simulink model "Lyapunov_3d"  (R2014a)
settings: Solver=ode45  StartTime=0.0  StopTime=100  RelTol=1e-3
values from neighbouring files (symbols this model uses):
  beta = 5    [lyapunov_vf.m]    (also in lyapunov_vf_3d.m; vector_cr_1.m)
  gam = 0.2    [lyapunov_vf.m]    (also in lyapunov_vf_3d.m; vector_cr_1.m)
  r = 20    [lsl.m]    (also in lyapunov_vf.m = 30; lyapunov_vf_3d.m = 100; rsl.m)
  vel = 10    [lyapunov_vf.m]    (also in lyapunov_vf_3d.m; vector_cr_1.m)
  x_int = -100    [lsl.m]    (also in lyapunov_vf.m; lyapunov_vf_3d.m = 20; rsl.m = -300; vf.m = 0)
  y_int = 10    [lsl.m]    (also in lyapunov_vf.m = -200; lyapunov_vf_3d.m = 20; rsl.m = 0; vf.m = -50)
  z_int = 10    [lyapunov_vf_3d.m]
settings Model: Creator=User  LastModifiedBy=User

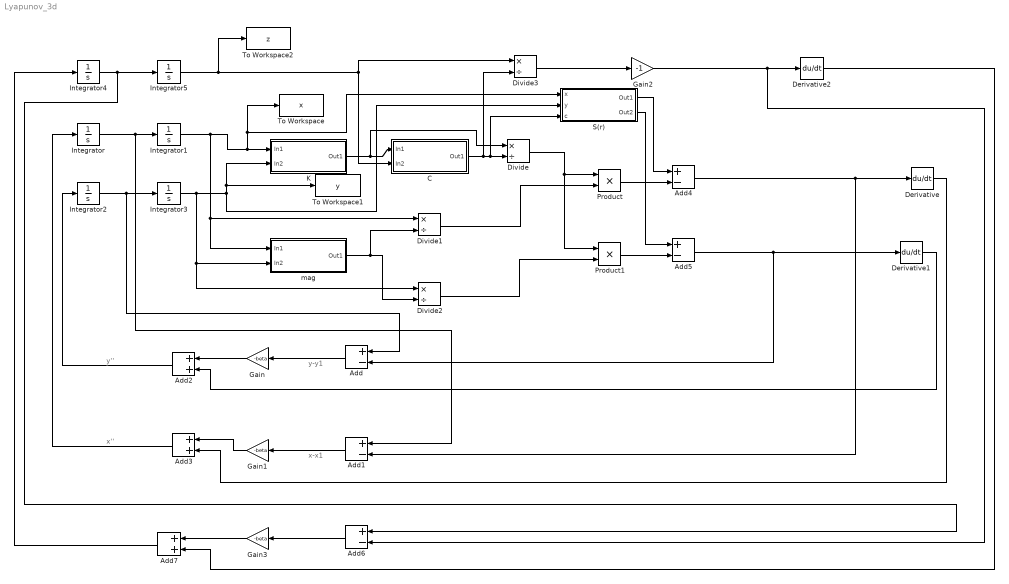
== system Lyapunov_3d ==
  note: y''
  note: x''
  note: x-x1
  note: y-y1
  Add{,1,4..6} (5 alike) : Sum  Inputs=+-
  Add2 : Sum
  Add3 : Sum
  Add7 : Sum
  C : Subsystem
  Derivative : Derivative
  Derivative1 : Derivative
  Derivative2 : Derivative
  Divide{,1..3} (4 alike) : Product  Inputs=*/
  Gain : Gain  Gain=-beta
  Gain1 : Gain  Gain=-beta
  Gain2 : Gain  Gain=-1
  Gain3 : Gain  Gain=-beta
  Integrator : Integrator
  Integrator1 : Integrator  InitialCondition=x_int
  Integrator2 : Integrator
  Integrator3 : Integrator  InitialCondition=y_int
  Integrator4 : Integrator
  Integrator5 : Integrator  InitialCondition=z_int
  K : Subsystem
  Product : Product
  Product1 : Product
  S(r) : Subsystem
  To Workspace : ToWorkspace  VariableName=x  SaveFormat=Timeseries  SampleTime=-1
  To Workspace1 : ToWorkspace  VariableName=y  SaveFormat=Timeseries  SampleTime=-1
  To Workspace2 : ToWorkspace  VariableName=z  SaveFormat=Timeseries  SampleTime=-1
  mag : Subsystem
  wires:
  Integrator1/1 -> Divide1/1, mag/1(In1), S(r)/1(x), To Workspace/1, K/1(In1)
  Integrator3/1 -> Divide2/1, mag/2(In2), K/2(In2), To Workspace1/1, S(r)/2(y)
  C/1(Out1) -> Divide3/2, S(r)/3(c), Divide/2
  K/1(Out1) -> Divide/1, C/1(In1)
  mag/1(Out1) -> Divide1/2, Divide2/2
  Divide/1 -> Product1/1, Product/1
  Divide1/1 -> Product/2
  Divide2/1 -> Product1/2
  Add/1 -> Gain/1
  Add1/1 -> Gain1/1
  Derivative1/1 -> Add2/2
  Gain/1 -> Add2/1
  Derivative/1 -> Add3/2
  Gain1/1 -> Add3/1
  Add2/1 -> Integrator2/1
  Add3/1 -> Integrator/1
  Add5/1 -> Derivative1/1, Add/2
  Product/1 -> Add4/2
  S(r)/1(Out1) -> Add4/1
  S(r)/2(Out2) -> Add5/1
  Product1/1 -> Add5/2
  Add4/1 -> Derivative/1, Add1/2
  Integrator/1 -> Add1/1, Integrator1/1
  Integrator2/1 -> Add/1, Integrator3/1
  Integrator4/1 -> Add6/1, Integrator5/1
  Integrator5/1 -> To Workspace2/1, C/2(In2), Divide3/1
  Divide3/1 -> Gain2/1
  Gain2/1 -> Add6/2, Derivative2/1
  Derivative2/1 -> Add7/2
  Add6/1 -> Gain3/1
  Gain3/1 -> Add7/1
  Add7/1 -> Integrator4/1

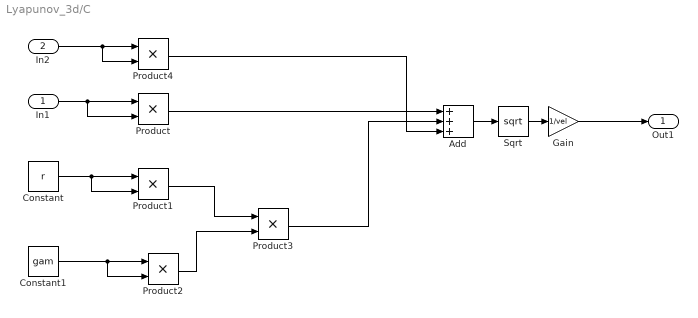
== system Lyapunov_3d/C ==
  In1 : Inport
  In2 : Inport  Port=2
  Add : Sum  Inputs=+++
  Constant : Constant  Value=r
  Constant1 : Constant  Value=gam
  Gain : Gain  Gain=1/vel
  Product{,1..4} (5 alike) : Product
  Sqrt : Sqrt  SaturateOnIntegerOverflow=on
  Out1 : Outport
  wires:
  Add/1 -> Sqrt/1
  Product/1 -> Add/1
  In1/1 -> Product/2, Product/1
  Constant/1 -> Product1/2, Product1/1
  Constant1/1 -> Product2/2, Product2/1
  Product1/1 -> Product3/1
  Product2/1 -> Product3/2
  Product3/1 -> Add/2
  Gain/1 -> Out1/1
  Sqrt/1 -> Gain/1
  In2/1 -> Product4/1, Product4/2
  Product4/1 -> Add/3

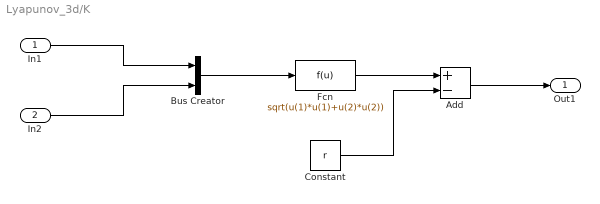
== system Lyapunov_3d/K ==
  In1 : Inport
  In2 : Inport  Port=2
  Add : Sum  Inputs=+-
  Bus Creator : BusCreator  Inputs=2
  Constant : Constant  Value=r
  Fcn : Fcn  Expr=sqrt(u(1)*u(1)+u(2)*u(2))
  Out1 : Outport
  wires:
  In2/1 -> Bus Creator/2
  In1/1 -> Bus Creator/1
  Bus Creator/1 -> Fcn/1
  Constant/1 -> Add/2
  Fcn/1 -> Add/1
  Add/1 -> Out1/1

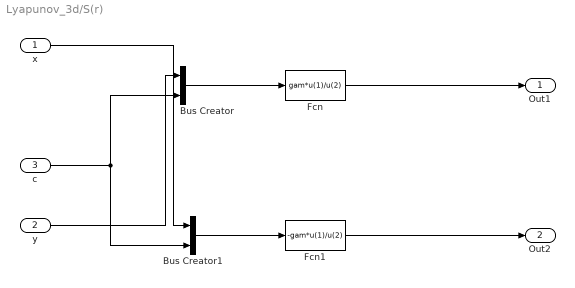
== system Lyapunov_3d/S(r) ==
  x : Inport
  y : Inport  Port=2
  c : Inport  Port=3
  Bus Creator : BusCreator  Inputs=2
  Bus Creator1 : BusCreator  Inputs=2
  Fcn : Fcn  Expr=gam*u(1)/u(2)
  Fcn1 : Fcn  Expr=-gam*u(1)/u(2)
  Out1 : Outport
  Out2 : Outport  Port=2
  wires:
  x/1 -> Bus Creator1/1
  c/1 -> Bus Creator/2, Bus Creator1/2
  Bus Creator/1 -> Fcn/1
  Fcn/1 -> Out1/1
  y/1 -> Bus Creator/1
  Bus Creator1/1 -> Fcn1/1
  Fcn1/1 -> Out2/1

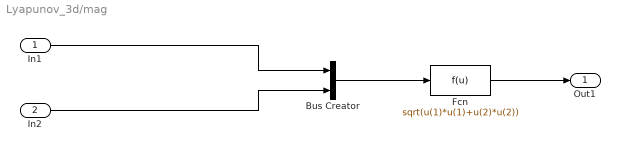
== system Lyapunov_3d/mag ==
  In1 : Inport
  In2 : Inport  Port=2
  Bus Creator : BusCreator  Inputs=2
  Fcn : Fcn  Expr=sqrt(u(1)*u(1)+u(2)*u(2))
  Out1 : Outport
  wires:
  In2/1 -> Bus Creator/2
  In1/1 -> Bus Creator/1
  Bus Creator/1 -> Fcn/1
  Fcn/1 -> Out1/1
